simulink model "PathUpdateObsAvoidDeerPoly"  (R2014b)
settings: Solver=ode45  SolverMode=SingleTasking  StartTime=0.0  StopTime=25  RelTol=1e-3
libraries: Solver_SF x1
settings Model: CovMetricSettings=dwe  CovHtmlReporting=off  covSaveCumulativeToWorkspaceVar=off  CovSaveSingleToWorkspaceVar=off  CovExternalEMLEnable=on  CovSFcnEnable=on  Creator=elowe  LastModifiedBy=mkhan
settings DataIOCC: LimitDataPoints=off  SaveFormat=StructureWithTime  ReturnWorkspaceOutputs=on
settings DebuggingCC: SolverPrmCheckMsg=none  FrameProcessingCompatibilityMsg=error  SFUnexpectedBacktrackingDiag=error  SFNoUnconditionalDefaultTransitionDiag=error
settings HardwareCC: ProdBitPerPointer=64  ProdLargestAtomicFloat=Float  ProdIntDivRoundTo=Zero  ProdEndianess=LittleEndian  ProdHWDeviceType=Specified
settings ModelReferenceCC: PropagateSignalLabelsOutOfModel=on
settings SFSimCC: SimUseLocalCustomCode=on
settings RTWCC: RTWUseLocalCustomCode=on
settings GRTTargetCC: TargetLangStandard=C99 (ISO)

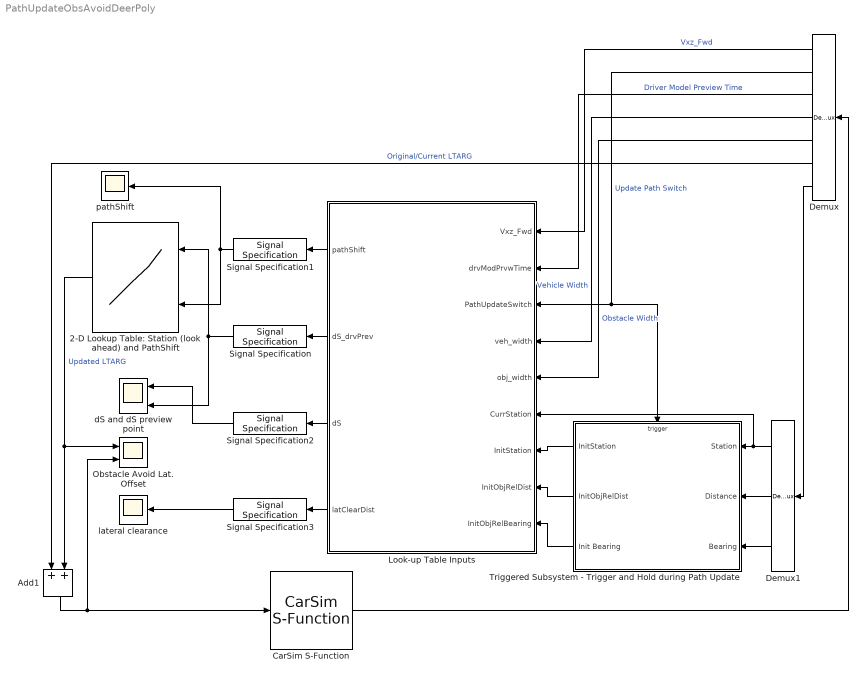
== system PathUpdateObsAvoidDeerPoly ==
  2-D Lookup Table: Station (look ahead) and PathShift : Lookup_n-D  BreakpointsForDimension1=|  BreakpointsForDimension2=|  Table=|  InternalRulePriority=Speed  RndMeth=Simplest  InputSameDT=on
      Table=|
      | [         0         0         0         0         0         0;
      |    -0.0420   -0.0250    0.0100    0.0350    0.0400    0.0630;
      |    -0.2430   -0.1430    0.0550    0.2060    0.2310    0.3660;
      |    -0.6380   -0.3750    0.1450    0.5400    0.6070    0.9580;
      |    -1.1770   -0.6930    0.2680    0.9980    1.1210    1.7640;
      |    -1.7660   -1.0410    0.4020    1.4980    1.6810    2.6420;
      |    -2.2960   -1.3540    0.5230    1.9470    2.1860    3.4320;
      |    -2.6740   -1.5760    0.6090    2.2670    2.5450    3.9990;
      |    -2.8570   -1.6840    0.6510    2.4220    2.7200    4.2760;
      |    -2.8900   -1.7030    0.6580    2.4500    2.7510    4.3250;
      |    -2.8900   -1.7000    0.6600    2.4500    2.7500    4.3250]
      BreakpointsForDimension1=|
      | [0    3.6805    7.3611   11.0416   14.7221   18.4027   22.0832   25.7637   29.4443   33.1248 40.49
      | ]
      BreakpointsForDimension2=|
      | [-2.89 -1.70 0.66 2.45 2.75	4.33
      | ]
  Add1 : Sum
  CarSim S-Function : Solver_SF/CarSim S-Function  Priority=1  SIMFILE=simfile.sim  Run_RTs=off  vs_state_ind=Run  StopMode_ind=Vehicle Model
  Demux : Demux  Outputs=[1 1 1 1 1 1 3]
  Demux1 : Demux  Outputs=3
  Look-up Table Inputs : MATLAB Function  TreatAsAtomicUnit=on
  Obstacle Avoid Lat. Offset : Scope  NumInputPorts=2
      settings: YMin=-8.2043~-5  YMax=3.67999~5
  Signal Specification{,1..3} (4 alike) : SignalSpecification  Dimensions=1
  Triggered Subsystem - Trigger and Hold during Path Update : Subsystem  TreatAsAtomicUnit=on
  dS and dS preview point : Scope  NumInputPorts=2
      settings: YMin=-3.25112~-5  YMax=69.51695~5
  lateral clearance : Scope
      settings: YMin=-1.09723  YMax=1.81193
  pathShift : Scope
      settings: YMin=-2.6654  YMax=4.25395  SaveName=ScopeData2
  wires:
  Demux/1 -> Look-up Table Inputs/1(Vxz_Fwd)  "Vxz_Fwd"
  CarSim S-Function/1 -> Demux/1
  Demux/7 -> Demux1/1
  Demux/6 -> Add1/1  "Original/Current LTARG"
  Demux1/1 -> Look-up Table Inputs/6(CurrStation), Triggered Subsystem - Trigger and Hold during Path Update/1(Station)
  Demux1/2 -> Triggered Subsystem - Trigger and Hold during Path Update/2(Distance)
  Demux1/3 -> Triggered Subsystem - Trigger and Hold during Path Update/3(Bearing)
  Demux/2 -> Triggered Subsystem - Trigger and Hold during Path Update/Trigger, Look-up Table Inputs/3(PathUpdateSwitch)  "Update Path Switch"
  Triggered Subsystem - Trigger and Hold during Path Update/2(InitObjRelDist) -> Look-up Table Inputs/8(InitObjRelDist)
  Triggered Subsystem - Trigger and Hold during Path Update/1(InitStation) -> Look-up Table Inputs/7(InitStation)
  Demux/3 -> Look-up Table Inputs/2(drvModPrvwTime)  "Driver Model Preview Time"
  Add1/1 -> CarSim S-Function/1, Obstacle Avoid Lat. Offset/2
  2-D Lookup Table: Station (look ahead) and PathShift/1 -> Add1/2, Obstacle Avoid Lat. Offset/1  "Updated LTARG"
  Demux/4 -> Look-up Table Inputs/4(veh_width)  "Vehicle Width"
  Demux/5 -> Look-up Table Inputs/5(obj_width)  "Obstacle Width"
  Triggered Subsystem - Trigger and Hold during Path Update/3(Init Bearing) -> Look-up Table Inputs/9(InitObjRelBearing)
  Look-up Table Inputs/1(pathShift) -> Signal Specification1/1
  Signal Specification1/1 -> 2-D Lookup Table: Station (look ahead) and PathShift/2, pathShift/1
  Look-up Table Inputs/2(dS_drvPrev) -> Signal Specification/1
  Signal Specification/1 -> 2-D Lookup Table: Station (look ahead) and PathShift/1, dS and dS preview point/2
  Look-up Table Inputs/3(dS) -> Signal Specification2/1
  Signal Specification2/1 -> dS and dS preview point/1
  Look-up Table Inputs/4(latClearDist) -> Signal Specification3/1
  Signal Specification3/1 -> lateral clearance/1

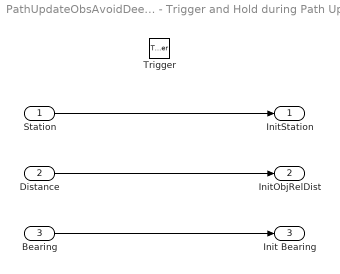
== system PathUpdateObsAvoidDeerPoly/Triggered Subsystem - Trigger and Hold during Path Update ==
  Station : Inport
  Distance : Inport  Port=2
  Bearing : Inport  Port=3
  Trigger : TriggerPort
  InitStation : Outport
  InitObjRelDist : Outport  Port=2
  Init Bearing : Outport  Port=3
  wires:
  Station/1 -> InitStation/1
  Distance/1 -> InitObjRelDist/1
  Bearing/1 -> Init Bearing/1

== matlab function PathUpdateObsAvoidDeerPoly/Look-up Table Inputs ==
  data: Vxz_Fwd input; drvModPrvwTime input; PathUpdateSwitch input; veh_width input; obj_width input; CurrStation input; pathShift output; dS_drvPrev output; dS output; latClearDist output; InitStation input; InitObjRelDist input; InitObjRelBearing input
function [pathShift, dS_drvPrev, dS, latClearDist] = ...
    LookUpTableInputs(Vxz_Fwd, drvModPrvwTime, PathUpdateSwitch, ...
    veh_width, obj_width, ...
    CurrStation, InitStation, InitObjRelDist, InitObjRelBearing)


% Vx_Fwd [km/h] simple translation of the vehicle x-velocity 
% PathUpdateSwitch [-] boolean flag noting when the path 
% should be updated, based on a threshold value in CarSim ( *** moved to 
% matlab later)
prevDist = (Vxz_Fwd/3.6)*drvModPrvwTime; % [m], the distance at which the 
% driver model preview point is located, in front of the vehicle's 
% origin. This is based on the curren vehicle speed and the designated 
% steerin conroller preview time TPREV 

% Only make updates to the path, if the path update flag is high
if (PathUpdateSwitch > 0)
    % calculate the differenc between the current/actual vehicle station
    % and the station at the exact time the path update process was
    % initiated 
    dS = CurrStation - InitStation;     
    dS_drvPrev = dS + prevDist; % [m] station at which the driver
    % model single preview point is located
    
    %convert the object relative bearing to radians
    InitObjRelBearingRad = InitObjRelBearing * pi / 180; % [rad]
    
    % relative obj. bearing threshold for determining left turn or right 
    % turn lane change maneuver. this value can vary depending on the type
    % of road sensed, or if snow/other debris is detected on the road 
    % surface vs. being clear and dry
    % Value = 0, means equal propensity to steer right vs. left if an
    % obstalce appears on the exact centerline of the ego vehicle's heading
    
    % Set this to 0.045 [rad] to achieve the same results as the Embedded
    % Python Example
    relBearRadThresh = 0.045; % [rad] 

    % the offset is the lateral relative distance from the current vehicle 
    % heading to the sensed object
        % it determines how far off-center the obstruction is located
        % the absolute value is used because the a bearing switching
        % if-statement determines which direction the ego vehicle steers 
        % for the maneuver 
    
    offset = InitObjRelDist*abs(sin(InitObjRelBearingRad)); 
    
    % tuning parameter for lateral clearance distance between vehcile and
    % obstacle
    latClearCoeff = 1.0; % [-] %1.125 will achieve the same 
    % vehicle-to-object spacing results as the Embedded Pythod example
    
    % in the short term, assume object width = 2
    % used to calculate clearance distances, below
    vehObjWidthSum = veh_width + obj_width;
    
    % pathShift is the peak latreal distance the steering controller should
    % aim to achive, during the maneuver    
    pathShift = latClearCoeff*(vehObjWidthSum) - offset;
    
    % lateral clearance distance is calculated peak lateral space between 
    % front left or write corner of the ego vehicle, and the side of 
    % the sensed object
    latClearDist = pathShift - 0.5*vehObjWidthSum; 
       
    % this if-statement determines if the the ego veh, goes left or right
    % during the avoidance maneuver
    % if the relative bearing between the ego vehicle and the sensed object
    % is greater than a specifed threshold, steer to the right, otherwise,
    % steer to the left, for the avoidance maneuver
    if (InitObjRelBearingRad > relBearRadThresh)
        pathShift = -pathShift; 
    end
else
    pathShift = 0; % [m]
    dS = 0;
    dS_drvPrev = 0;
    latClearDist = 0; 
end
